simulink subsystem "analog_inputs"  (R2022b)
settings: Solver=VariableStepAuto  StartTime=0.0  StopTime=10.0  RelTol=1e-3
libraries: wheels x7, pot_test x1, brake x1, throttle x1
settings Model: Creator=serga  LastModifiedBy=serga

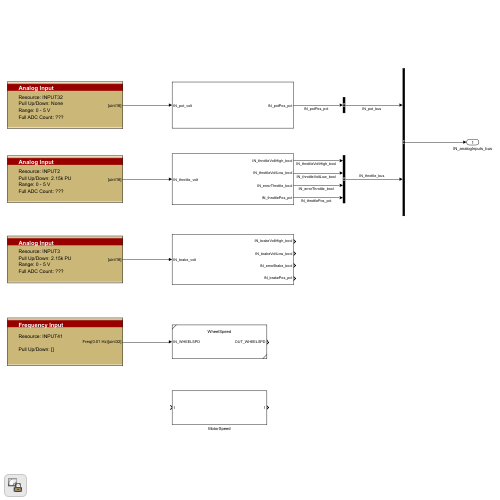
[thumbnail: Simulink's stored preview of the top-level diagram]
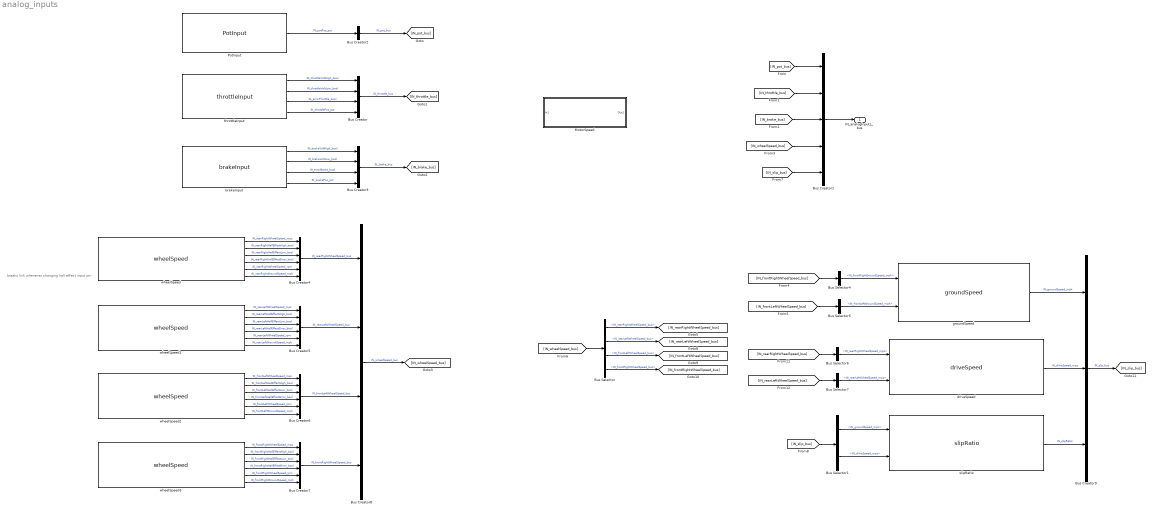
== system analog_inputs ==
  note: breaks link whenever changing hall effect input pin
  Bus Creator : BusCreator  Inputs=4
  Bus Creator1 : BusCreator  Inputs=5
  Bus Creator2 : BusCreator  Inputs=1
  Bus Creator3 : BusCreator  Inputs=4
  Bus Creator{4..7} (4 alike) : BusCreator  Inputs=6
  Bus Creator8 : BusCreator  Inputs=4
  Bus Creator9 : BusCreator  Inputs=3
  Bus Selector : BusSelector  OutputSignals=IN_rearRightWheelSpeed_bus,IN_rearLeftWheelSpeed_bus,IN_frontLeftWheelSpeed_bus,IN_frontRightWheelSpeed_bus
  Bus Selector1 : BusSelector  OutputSignals=IN_groundSpeed_mph,IN_driveSpeed_mps
  Bus Selector4 : BusSelector  OutputSignals=IN_frontRightGroundSpeed_mph
  Bus Selector5 : BusSelector  OutputSignals=IN_frontLeftGroundSpeed_mph
  Bus Selector6 : BusSelector  OutputSignals=IN_rearRightWheelSpeed_mps
  Bus Selector7 : BusSelector  OutputSignals=IN_rearLeftWheelSpeed_mps
  MotorSpeed : Subsystem
  PotInput : pot_test/PotInput  SystemSampleTime=-1  VariantActivationTime=update diagram  Latency=0  AutoFrameSizeCalculation=off
  brakeInput : brake/brakeInput  SystemSampleTime=-1  VariantActivationTime=update diagram  Latency=0  AutoFrameSizeCalculation=off
  driveSpeed : wheels/driveSpeed  SystemSampleTime=-1  VariantActivationTime=update diagram  Latency=0  AutoFrameSizeCalculation=off
  groundSpeed : wheels/groundSpeed  SystemSampleTime=-1  VariantActivationTime=update diagram  Latency=0  AutoFrameSizeCalculation=off
  slipRatio : wheels/slipRatio  SystemSampleTime=-1  VariantActivationTime=update diagram  Latency=0  AutoFrameSizeCalculation=off
  throttleInput : throttle/throttleInput  SystemSampleTime=-1  VariantActivationTime=update diagram  Latency=0  AutoFrameSizeCalculation=off
  wheelSpeed : wheels/wheelSpeed  pos='rearRight'
  wheelSpeed1 : wheels/wheelSpeed  pos='rearLeft'
  wheelSpeed2 : wheels/wheelSpeed  pos='frontLeft'
  wheelSpeed3 : wheels/wheelSpeed  pos='frontRight'
  IN_analogInputs_bus : Outport
  wires:
  throttleInput/1 -> Bus Creator/1  "IN_throttleVoltHigh_bool"
  throttleInput/2 -> Bus Creator/2  "IN_throttleVoltLow_bool"
  throttleInput/3 -> Bus Creator/3  "IN_errorThrottle_bool"
  throttleInput/4 -> Bus Creator/4  "IN_throttlePos_pct"
  Bus Creator1/1 -> IN_analogInputs_bus/1
  PotInput/1 -> Bus Creator2/1  "IN_potPos_pct"
  brakeInput/1 -> Bus Creator3/1  "IN_brakeVoltHigh_bool"
  brakeInput/2 -> Bus Creator3/2  "IN_brakeVoltLow_bool"
  brakeInput/3 -> Bus Creator3/3  "IN_errorBrake_bool"
  brakeInput/4 -> Bus Creator3/4  "IN_brakePos_pct"
  wheelSpeed/1 -> Bus Creator4/1  "IN_rearRightWheelSpeed_mps"
  wheelSpeed/2 -> Bus Creator4/2  "IN_rearRightHallEffectHigh_bool"
  wheelSpeed/3 -> Bus Creator4/3  "IN_rearRightHallEffectLow_bool"
  wheelSpeed/4 -> Bus Creator4/4  "IN_rearRightHallEffectError_bool"
  wheelSpeed/5 -> Bus Creator4/5  "IN_rearRightWheelSpeed_rpm"
  wheelSpeed1/1 -> Bus Creator5/1  "IN_rearLeftWheelSpeed_mps"
  wheelSpeed1/2 -> Bus Creator5/2  "IN_rearLeftHallEffectHigh_bool"
  wheelSpeed1/3 -> Bus Creator5/3  "IN_rearLeftHallEffectLow_bool"
  wheelSpeed1/4 -> Bus Creator5/4  "IN_rearLeftHallEffectError_bool"
  wheelSpeed1/5 -> Bus Creator5/5  "IN_rearLeftWheelSpeed_rpm"
  wheelSpeed2/1 -> Bus Creator6/1  "IN_frontLeftWheelSpeed_mps"
  wheelSpeed2/2 -> Bus Creator6/2  "IN_frontLeftHallEffectHigh_bool"
  wheelSpeed2/3 -> Bus Creator6/3  "IN_frontLeftHallEffectLow_bool"
  wheelSpeed2/4 -> Bus Creator6/4  "IN_frontLeftHallEffectError_bool"
  wheelSpeed2/5 -> Bus Creator6/5  "IN_frontLeftWheelSpeed_rpm"
  wheelSpeed3/1 -> Bus Creator7/1  "IN_frontRightWheelSpeed_mps"
  wheelSpeed3/2 -> Bus Creator7/2  "IN_frontRightHallEffectHigh_bool"
  wheelSpeed3/3 -> Bus Creator7/3  "IN_frontRightHallEffectLow_bool"
  wheelSpeed3/4 -> Bus Creator7/4  "IN_frontRightHallEffectError_bool"
  wheelSpeed3/5 -> Bus Creator7/5  "IN_frontRightWheelSpeed_rpm"
  wheelSpeed2/6 -> Bus Creator6/6  "IN_frontLeftGroundSpeed_mph"
  wheelSpeed3/6 -> Bus Creator7/6  "IN_frontRightGroundSpeed_mph"
  Bus Creator2/1 -> [IN_pot_bus]  "IN_pot_bus"
  Bus Creator/1 -> [IN_throttle_bus]  "IN_throttle_bus"
  Bus Creator3/1 -> [IN_brake_bus]  "IN_brake_bus"
  Bus Creator4/1 -> Bus Creator8/1  "IN_rearRightWheelSpeed_bus"
  Bus Creator5/1 -> Bus Creator8/2  "IN_rearLeftWheelSpeed_bus"
  Bus Creator6/1 -> Bus Creator8/3  "IN_frontLeftWheelSpeed_bus"
  Bus Creator7/1 -> Bus Creator8/4  "IN_frontRightWheelSpeed_bus"
  [IN_pot_bus] -> Bus Creator1/1
  [IN_throttle_bus] -> Bus Creator1/2
  [IN_brake_bus] -> Bus Creator1/3
  wheelSpeed/6 -> Bus Creator4/6  "IN_rearRightGroundSpeed_mph"
  wheelSpeed1/6 -> Bus Creator5/6  "IN_rearLeftGroundSpeed_mph"
  Bus Creator8/1 -> [IN_wheelSpeed_bus]  "IN_wheelSpeed_bus"
  [IN_wheelSpeed_bus] -> Bus Creator1/4
  [IN_rearLeftWheelSpeed_bus] -> Bus Selector7/1
  driveSpeed/1 -> Bus Creator9/2  "IN_driveSpeed_mps"
  Bus Selector6/1 -> driveSpeed/1  "<IN_rearRightWheelSpeed_mps>"
  Bus Selector7/1 -> driveSpeed/2  "<IN_rearLeftWheelSpeed_mps>"
  [IN_frontRightWheelSpeed_bus] -> Bus Selector4/1
  Bus Selector1/2 -> slipRatio/2  "<IN_driveSpeed_mps>"
  Bus Selector4/1 -> groundSpeed/1  "<IN_frontRightGroundSpeed_mph>"
  [IN_frontLeftWheelSpeed_bus] -> Bus Selector5/1
  slipRatio/1 -> Bus Creator9/3  "IN_slipRatio"
  Bus Selector1/1 -> slipRatio/1  "<IN_groundSpeed_mph>"
  groundSpeed/1 -> Bus Creator9/1  "IN_groundSpeed_mph"
  Bus Selector5/1 -> groundSpeed/2  "<IN_frontLeftGroundSpeed_mph>"
  [IN_rearRightWheelSpeed_bus] -> Bus Selector6/1
  [IN_wheelSpeed_bus] -> Bus Selector/1
  Bus Selector/1 -> [IN_rearRightWheelSpeed_bus]  "<IN_rearRightWheelSpeed_bus>"
  Bus Selector/2 -> [IN_rearLeftWheelSpeed_bus]  "<IN_rearLeftWheelSpeed_bus>"
  Bus Selector/3 -> [IN_frontLeftWheelSpeed_bus]  "<IN_frontLeftWheelSpeed_bus>"
  Bus Selector/4 -> [IN_frontRightWheelSpeed_bus]  "<IN_frontRightWheelSpeed_bus>"
  Bus Creator9/1 -> [IN_slip_bus]  "IN_slip_bus"
  [IN_slip_bus] -> Bus Creator1/5
  [IN_slip_bus] -> Bus Selector1/1

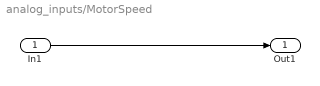
== system analog_inputs/MotorSpeed ==
  In1 : Inport
  Out1 : Outport
  wires:
  In1/1 -> Out1/1
